simulink model "joinX_1"  (R2021a)
settings: Solver=FixedStepAuto  StartTime=0.0  StopTime=10.0  RelTol=1e-3  EnableMultiTasking=on
settings Model: DataDictionary=worldDD.sldd  SILPILModeSetting=veronly  ExtModeTrigDuration=2  Creator=Koorosh  LastModifiedBy=Koorosh
settings OptimizationCC: EnhancedBackFolding=on  PassReuseOutputArgsAs=Individual arguments  ZeroExternalMemoryAtStartup=off  ZeroInternalMemoryAtStartup=off  MaxStackSize=64  OptimizeBlockOrder=speed  DifferentSizesBufferReuse=on  OptimizationCustomize=off  EfficientTunableParamExpr=on
settings DebuggingCC: ParameterTunabilityLossMsg=error
settings HardwareCC: ProdBitPerInt=16  ProdBitPerPointer=16  ProdBitPerSizeT=16  ProdBitPerPtrDiffT=16  ProdLargestAtomicFloat=None  ProdWordSize=8  ProdHWDeviceType=Atmel->AVR
settings SFSimCC: MATLABDynamicMemAlloc=off
settings RTWCC: SystemTargetFile=ert.tlc  HardwareBoard=Arduino Uno  TemplateMakefile=ert_default_tmf  Toolchain=Arduino AVR  BuildConfiguration=Faster Runs
settings CodeAppCC: ForceParamTrailComments=on  IgnoreCustomStorageClasses=off  OperatorAnnotations=on  SimulinkDataObjDesc=on  SFDataObjDesc=on  InsertBlockDesc=on
settings ERTTargetCC: SupportContinuousTime=on  SupportVariableSizeSignals=on  ExtModeStaticAllocSize=250

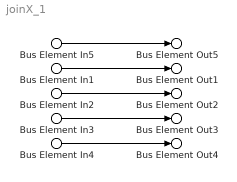
== system joinX_1 ==
  Bus Element In5 : Inport  PortName=u
  Bus Element In1 : Inport  Port=2  PortName=x1
  Bus Element In2 : Inport  Port=3  PortName=x2
  Bus Element In3 : Inport  Port=4  PortName=x3
  Bus Element In4 : Inport  Port=5  PortName=x4
  Bus Element Out5 : Outport  PortName=X  Element=u
  Bus Element Out1 : Outport  PortName=X  Element=x1
  Bus Element Out2 : Outport  PortName=X  Element=x2
  Bus Element Out3 : Outport  PortName=X  Element=x3
  Bus Element Out4 : Outport  PortName=X  Element=x4
  wires:
  Bus Element In1/1 -> Bus Element Out1/1
  Bus Element In2/1 -> Bus Element Out2/1
  Bus Element In3/1 -> Bus Element Out3/1
  Bus Element In4/1 -> Bus Element Out4/1
  Bus Element In5/1 -> Bus Element Out5/1
